simulink model "SA_ACex4_ZADANIE3_2_MODEL"  (Simulink 9.1)
settings: Solver=VariableStepAuto  StartTime=0.0  StopTime=80  FixedStep=0.01  MaxStep=0.01  RelTol=1e-3  EnableMultiTasking=on
values from neighbouring files (symbols this model uses):
  omega_r = 0.25    [SA_ACex4_SKRYPT.m]
  sigma2e = 0.0    (= 0)    [SA_ACex4_SKRYPT.m]
  Ta = 0.005    [SA_ACex4_SKRYPT.m]
  Tc = 0.001    [SA_ACex4_SKRYPT.m]
  TF = 1.5*Ta    (= 0.0075)    [SA_ACex4_SKRYPT.m]
  Yr = 0.15    [SA_ACex4_SKRYPT.m]
libraries: simulink x1
settings Model: Creator=Gebruiker  LastModifiedBy=szymon
settings DataIOCC: LimitDataPoints=on  SignalLoggingSaveFormat=ModelDataLogs
settings OptimizationCC: InitFltsAndDblsToZero=on
settings DebuggingCC: SaveWithParameterizedLinksMsg=none  SignalResolutionControl=TryResolveAllWithWarning  SolverPrmCheckMsg=warning  MultiTaskDSMMsg=warning  MultiTaskCondExecSysMsg=none  FcnCallInpInsideContextMsg=warning
settings SFSimCC: SimUseLocalCustomCode=on
settings RTWCC: RTWUseLocalCustomCode=on
settings GRTTargetCC: TargetFcnLib=ansi_tfl_tmw.mat
settings ConfigComp: CovExternalEMLEnable=on

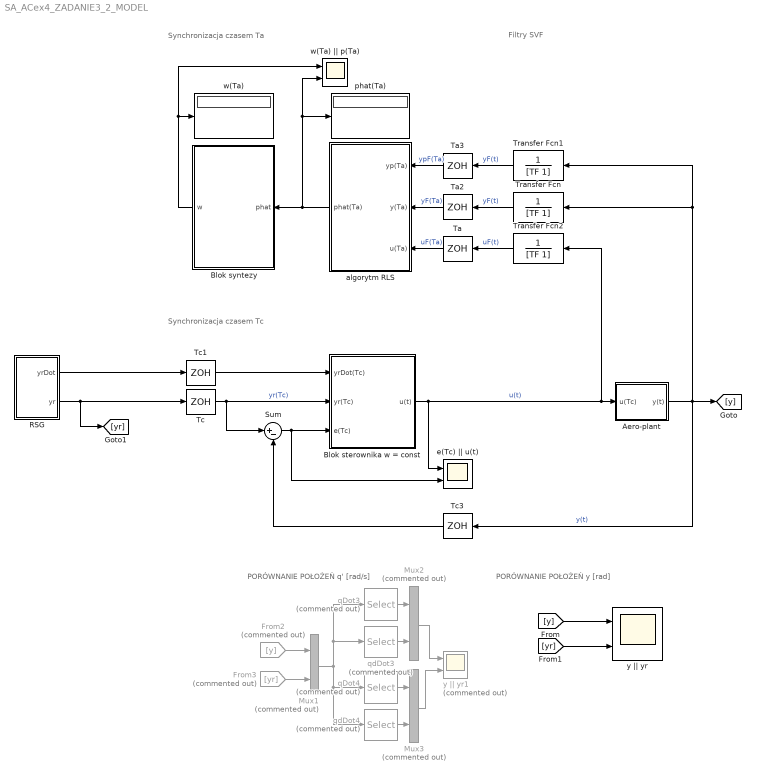
== system SA_ACex4_ZADANIE3_2_MODEL ==
  note: Synchronizacja czasem Ta
  note: Filtry SVF
  note: PORÓWNANIE POŁOŻEŃ
      | y [rad]
  note: Synchronizacja czasem Tc
  note: PORÓWNANIE POŁOŻEŃ
      | q' [rad/s]
  Aero-plant : Subsystem
  Blok sterownika w = const : Subsystem
  Blok syntezy : Subsystem
  From2 : From  Commented=on  GotoTag=y
  From3 : From  Commented=on  GotoTag=yr
  Mux1 : Mux  Commented=on  Inputs=2
  Mux2 : Mux  Commented=on  Inputs=2
  Mux3 : Mux  Commented=on  Inputs=2
  RSG : Subsystem
  Sum : Sum  Inputs=|+-
  Ta : ZeroOrderHold  SampleTime=Ta
  Ta2 : ZeroOrderHold  SampleTime=Ta
  Ta3 : ZeroOrderHold  SampleTime=Ta
  Tc : ZeroOrderHold  SampleTime=Tc
  Tc1 : ZeroOrderHold  SampleTime=Tc
  Tc3 : ZeroOrderHold  SampleTime=Tc
  Transfer Fcn : TransferFcn  Numerator=[0 1]  Denominator=[TF 1]
  Transfer Fcn1 : TransferFcn  Numerator=[0 1]  Denominator=[TF 1]
  Transfer Fcn2 : TransferFcn  Numerator=[0 1]  Denominator=[TF 1]
  algorytm RLS : Subsystem
  e(Tc) || u(t) : Scope  NumInputPorts=2
  phat(Ta) : Display
  qDot3 : Selector  Commented=on  InputPortWidth=4  IndexOptions=Index vector (dialog)  Indices=[1]  OutputSizes=1
  qDot4 : Selector  Commented=on  InputPortWidth=4  IndexOptions=Index vector (dialog)  Indices=[2]  OutputSizes=1
  qdDot3 : Selector  Commented=on  InputPortWidth=4  IndexOptions=Index vector (dialog)  Indices=[3]  OutputSizes=1
  qdDot4 : Selector  Commented=on  InputPortWidth=4  IndexOptions=Index vector (dialog)  Indices=[4]  OutputSizes=1
  w(Ta) : Display
  w(Ta) || p(Ta) : Scope  NumInputPorts=2
  y || yr : Scope  NumInputPorts=2
  y || yr1 : Scope  Commented=on  NumInputPorts=2
  wires:
  Aero-plant/1(y(t)) -> Transfer Fcn1/1, Transfer Fcn/1, [y], Tc3/1  "y(t)"
  RSG/1(yrDot) -> Tc1/1
  RSG/2(yr) -> [yr], Tc/1
  Tc/1 -> Sum/1, Blok sterownika w = const/2(yr(Tc))  "yr(Tc)"
  Blok sterownika w = const/1(u(t)) -> e(Tc) || u(t)/1, Transfer Fcn2/1, Aero-plant/1(u(Tc))  "u(t)"
  Transfer Fcn1/1 -> Ta3/1  "yF(t)"
  Transfer Fcn2/1 -> Ta/1  "uF(t)"
  Transfer Fcn/1 -> Ta2/1  "yF(t)"
  Ta/1 -> algorytm RLS/3(u(Ta))  "uF(Ta)"
  Ta2/1 -> algorytm RLS/2(y(Ta))  "yF(Ta)"
  Ta3/1 -> algorytm RLS/1(yp(Ta))  "ypF(Ta)"
  Blok syntezy/1(w) -> w(Ta) || p(Ta)/1, w(Ta)/1
  algorytm RLS/1(phat(Ta)) -> phat(Ta)/1, w(Ta) || p(Ta)/2, Blok syntezy/1(phat)
  Tc1/1 -> Blok sterownika w = const/1(yrDot(Tc))
  Sum/1 -> e(Tc) || u(t)/2, Blok sterownika w = const/3(e(Tc))
  [yr] -> y || yr/2
  [y] -> y || yr/1
  Tc3/1 -> Sum/2
  Mux3/1 -> y || yr1/2
  Mux2/1 -> y || yr1/1
  From3/1 -> Mux1/2
  qdDot3/1 -> Mux2/2
  Mux1/1 -> qdDot4/1, qDot4/1, qdDot3/1, qDot3/1
  qdDot4/1 -> Mux3/2
  qDot3/1 -> Mux2/1
  qDot4/1 -> Mux3/1
  From2/1 -> Mux1/1

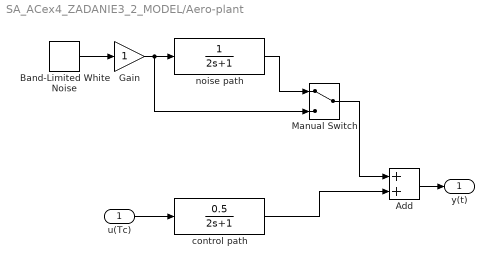
== system SA_ACex4_ZADANIE3_2_MODEL/Aero-plant ==
  u(Tc) : Inport
  Add : Sum
  Band-Limited White Noise : simulink/Sources/Band-Limited White Noise  Cov=[sigma2e*Tc]  Ts=Tc  seed=[23341]
  Gain : Gain
  Manual Switch : ManualSwitch
  control path : TransferFcn  Numerator=[0.5]  Denominator=[2 1]
  noise path : TransferFcn  Denominator=[2 1]
  y(t) : Outport
  wires:
  control path/1 -> Add/2
  Band-Limited White Noise/1 -> Gain/1
  Gain/1 -> Manual Switch/2, noise path/1
  Add/1 -> y(t)/1
  u(Tc)/1 -> control path/1
  noise path/1 -> Manual Switch/1
  Manual Switch/1 -> Add/1

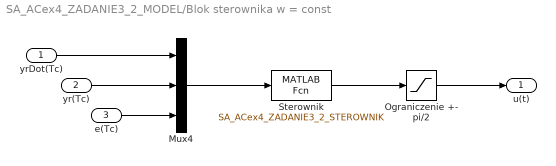
== system SA_ACex4_ZADANIE3_2_MODEL/Blok sterownika w = const ==
  yrDot(Tc) : Inport
  yr(Tc) : Inport  Port=2
  e(Tc) : Inport  Port=3
  Mux4 : Mux  Inputs=3
  Ograniczenie +- pi/2 : Saturate  UpperLimit=pi/2  LowerLimit=-pi/2
  Sterownik : MATLABFcn  MATLABFcn=SA_ACex4_ZADANIE3_2_STEROWNIK  OutputDimensions=1
  u(t) : Outport
  wires:
  Sterownik/1 -> Ograniczenie +- pi/2/1
  Ograniczenie +- pi/2/1 -> u(t)/1
  Mux4/1 -> Sterownik/1
  e(Tc)/1 -> Mux4/3
  yrDot(Tc)/1 -> Mux4/1
  yr(Tc)/1 -> Mux4/2

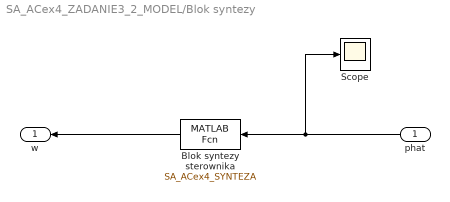
== system SA_ACex4_ZADANIE3_2_MODEL/Blok syntezy ==
  phat : Inport
  Blok syntezy sterownika : MATLABFcn  MATLABFcn=SA_ACex4_SYNTEZA
  Scope : Scope
  w : Outport
  wires:
  phat/1 -> Scope/1, Blok syntezy sterownika/1
  Blok syntezy sterownika/1 -> w/1

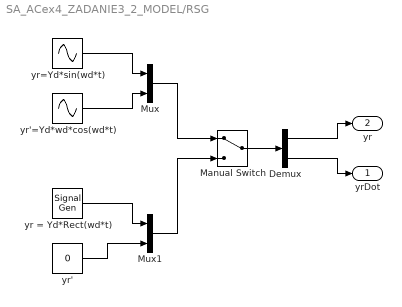
== system SA_ACex4_ZADANIE3_2_MODEL/RSG ==
  Demux : Demux  Outputs=2
  Manual Switch : ManualSwitch
  Mux : Mux  Inputs=2
  Mux1 : Mux  Inputs=2
  yr = Yd*Rect(wd*t) : SignalGenerator  WaveForm=square  Amplitude=Yr  Frequency=omega_r  Units=rad/sec
  yr' : Constant  Value=0
  yr'=Yd*wd*cos(wd*t) : Sin  Amplitude=Yr*omega_r  Frequency=omega_r  Phase=pi/2  SampleTime=0
  yr=Yd*sin(wd*t) : Sin  Amplitude=Yr  Frequency=omega_r  SampleTime=0
  yrDot : Outport
  yr : Outport  Port=2
  wires:
  yr=Yd*sin(wd*t)/1 -> Mux/1
  yr'=Yd*wd*cos(wd*t)/1 -> Mux/2
  yr = Yd*Rect(wd*t)/1 -> Mux1/1
  yr'/1 -> Mux1/2
  Mux/1 -> Manual Switch/1
  Mux1/1 -> Manual Switch/2
  Manual Switch/1 -> Demux/1
  Demux/1 -> yr/1
  Demux/2 -> yrDot/1

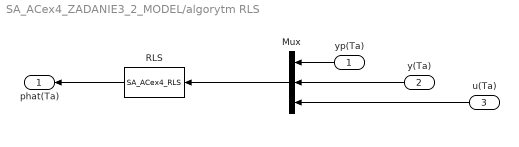
== system SA_ACex4_ZADANIE3_2_MODEL/algorytm RLS ==
  yp(Ta) : Inport
  y(Ta) : Inport  Port=2
  u(Ta) : Inport  Port=3
  Mux : Mux  Inputs=3
  RLS : MATLABFcn  MATLABFcn=SA_ACex4_RLS  OutputDimensions=2
  phat(Ta) : Outport
  wires:
  Mux/1 -> RLS/1
  RLS/1 -> phat(Ta)/1
  u(Ta)/1 -> Mux/3
  y(Ta)/1 -> Mux/2
  yp(Ta)/1 -> Mux/1
